simulink model "modela13"  (R2018b)
settings: Solver=VariableStepAuto  StartTime=0.0  StopTime=10.0  RelTol=1e-3
libraries: powerlib x39
settings Model: Creator=HP  LastModifiedBy=HP

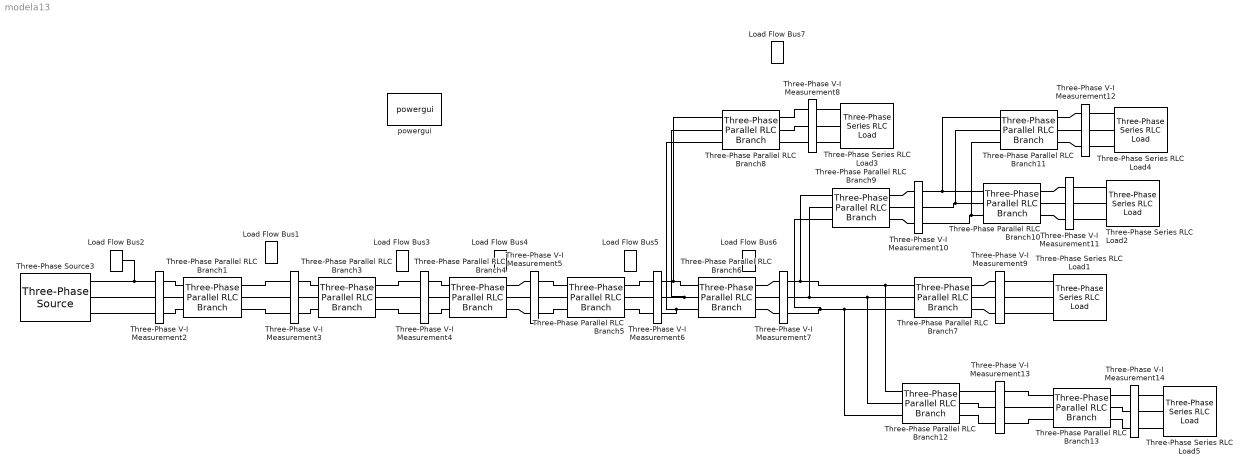
== system modela13 ==
  Load Flow Bus{1..7} (7 alike) : powerlib/Measurements/Load Flow Bus  LConnTagsString=a  Phases=single  Connectors=on one side  ID=BUS_1  Vbase=25e3  Vref=1.06  Vangle=0  VLF=1  VLFb=1  VLFc=1  angleLF=0  angleLFb=0  angleLFc=0
      settings: SourceProductName=Simscape Power Systems
  Three-Phase Parallel RLC Branch{1,3..13} (12 alike) : powerlib/Elements/Three-Phase Parallel RLC Branch  LConnTagsString=A|B|C  RConnTagsString=A|B|C  BranchType=RL  Resistance=6  Inductance=1.9e-3  Capacitance=1e-6  Measurements=None
      settings: SourceProductName=Simscape Power Systems  SourceProductBaseCode=PS
  Three-Phase Series RLC Load{1..5} (5 alike) : powerlib/Elements/Three-Phase Series RLC Load  LConnTagsString=A|B|C  Configuration=Y (grounded)  NominalVoltage=1000  Vabc=[1e3 1e3 1e3]  Vabcp=[1e3 1e3 1e3]  NominalFrequency=60  UnbalancedPower=off  ActivePower=20e6  InductivePower=10e6  CapacitivePower=0  Pabc=[10e3 9e3 11e3]  QLabc=[100 90 110]  QCabc=[100 90 110]  Pabcp=[10e3 9e3 11e3]  QLabcp=[100 90 110]  QCabcp=[100 90 110]  Measurements=None  LoadType=constant Z
  Three-Phase V-I Measurement{2..14} (13 alike) : powerlib/Measurements/Three-Phase V-I Measurement  VoltageMeasurement=no  SetLabelV=off  LabelV=Vabc  Vpu=off  VpuLL=off  CurrentMeasurement=no  SetLabelI=off  LabelI=Iabc  Ipu=off  Pbase=100e6  Vbase=500e3  OutputType=Complex  PhasorSimulation=off  PSBequivalent=0
  Three-Phase Source3 : powerlib/Electrical Sources/Three-Phase Source  InternalConnection=Yg  VoltagePhases=off  Voltage=25e3  PhaseAngle=0  Voltage_phases=[25e3 25e3 25e3]/sqrt(3)  PhaseAngles_phases=[0 -120 +120]  Frequency=50  NonIdealSource=on  SpecifyImpedance=on  Resistance=0.8929  Inductance=16.58e-3  ShortCircuitLevel=100e6  BaseVoltage=25e3  XRratio=7  BusType=swing  Pref=10e3  Qref=0  Prefabc=[10e3, 10e3, 10e3]  Qrefabc=[0, 0, 0]  Qmin=-inf  Qmax=inf
  powergui : powerlib/powergui  Priority=1  SimulationMode=Continuous  SampleTime=50e-6  frequency=60  Iterations=50  frequencyindice=50  Pbase=100e6  ErrMax=1e-4  UnitsV=kV  UnitsW=MW  buscounter=0  FunctionMessages=off  echomessages=off  EnableUseOfTLC=off  CurrentSourceSwitches=off  DisableSnubberDevices=off  DisableRonSwitches=off  DisableVfSwitches=off  DisplayEquations=off  SolverType=Tustin/Backward Euler (TBE)  Interpol=off  ExternalGateDelay=off  methode=off  Ts=100  x0status=blocks  SPID=off  SwTol=0  HookPort=off  RestoreLinks=warning  ResistiveCurrentMeasurement=off  Frange=[0:2:500]  Ylog=off  Xlog=on  ShowGrid=off  save=off  variable=ZData  structure=0  ZoomFFT=off  StartTime=0.0  cycles=1  DisplayStyle=1  fundamental=60  FreqAxis=off  MaxFrequency=1000  frequencyindicesteady=1  RmsSteady=1  display=off
  connections:
  Three-Phase V-I Measurement2/LConn2 -- Three-Phase Parallel RLC Branch1/RConn2
  Three-Phase V-I Measurement2/RConn3 -- Load Flow Bus2/LConn1 -- Three-Phase Source3/RConn3
  Three-Phase V-I Measurement2/RConn2 -- Three-Phase Source3/RConn2
  Three-Phase V-I Measurement2/RConn1 -- Three-Phase Source3/RConn1
  Three-Phase V-I Measurement2/LConn3 -- Three-Phase Parallel RLC Branch1/RConn1
  Three-Phase V-I Measurement2/LConn1 -- Three-Phase Parallel RLC Branch1/RConn3
  Three-Phase V-I Measurement3/LConn3 -- Three-Phase Parallel RLC Branch3/RConn1
  Three-Phase V-I Measurement3/LConn1 -- Three-Phase Parallel RLC Branch3/RConn3
  Three-Phase V-I Measurement3/LConn2 -- Three-Phase Parallel RLC Branch3/RConn2
  Three-Phase Parallel RLC Branch1/LConn1 -- Three-Phase V-I Measurement3/RConn3
  Three-Phase Parallel RLC Branch1/LConn2 -- Three-Phase V-I Measurement3/RConn2
  Three-Phase Parallel RLC Branch1/LConn3 -- Three-Phase V-I Measurement3/RConn1
  Three-Phase V-I Measurement4/LConn3 -- Three-Phase Parallel RLC Branch4/RConn1
  Three-Phase V-I Measurement4/LConn1 -- Three-Phase Parallel RLC Branch4/RConn3
  Three-Phase V-I Measurement4/LConn2 -- Three-Phase Parallel RLC Branch4/RConn2
  Three-Phase Parallel RLC Branch3/LConn1 -- Three-Phase V-I Measurement4/RConn3
  Three-Phase Parallel RLC Branch3/LConn2 -- Three-Phase V-I Measurement4/RConn2
  Three-Phase Parallel RLC Branch3/LConn3 -- Three-Phase V-I Measurement4/RConn1
  Three-Phase V-I Measurement5/LConn3 -- Three-Phase Parallel RLC Branch5/RConn1
  Three-Phase V-I Measurement5/LConn1 -- Three-Phase Parallel RLC Branch5/RConn3
  Three-Phase V-I Measurement5/LConn2 -- Three-Phase Parallel RLC Branch5/RConn2
  Three-Phase Parallel RLC Branch4/LConn1 -- Three-Phase V-I Measurement5/RConn3
  Three-Phase Parallel RLC Branch4/LConn2 -- Three-Phase V-I Measurement5/RConn2
  Three-Phase Parallel RLC Branch4/LConn3 -- Three-Phase V-I Measurement5/RConn1
  Three-Phase V-I Measurement6/LConn3 -- Three-Phase Parallel RLC Branch8/RConn1 -- Three-Phase Parallel RLC Branch6/RConn1
  Three-Phase V-I Measurement6/LConn1 -- Three-Phase Parallel RLC Branch6/RConn3 -- Three-Phase Parallel RLC Branch8/RConn3
  Three-Phase V-I Measurement6/LConn2 -- Three-Phase Parallel RLC Branch8/RConn2 -- Three-Phase Parallel RLC Branch6/RConn2
  Three-Phase Parallel RLC Branch5/LConn1 -- Three-Phase V-I Measurement6/RConn3
  Three-Phase Parallel RLC Branch5/LConn2 -- Three-Phase V-I Measurement6/RConn2
  Three-Phase Parallel RLC Branch5/LConn3 -- Three-Phase V-I Measurement6/RConn1
  Three-Phase V-I Measurement7/LConn3 -- Three-Phase Parallel RLC Branch9/RConn1 -- Three-Phase Parallel RLC Branch12/RConn1 -- Three-Phase Parallel RLC Branch7/RConn1
  Three-Phase V-I Measurement7/LConn1 -- Three-Phase Parallel RLC Branch9/RConn3 -- Three-Phase Parallel RLC Branch12/RConn3 -- Three-Phase Parallel RLC Branch7/RConn3
  Three-Phase V-I Measurement7/LConn2 -- Three-Phase Parallel RLC Branch9/RConn2 -- Three-Phase Parallel RLC Branch12/RConn2 -- Three-Phase Parallel RLC Branch7/RConn2
  Three-Phase Parallel RLC Branch6/LConn1 -- Three-Phase V-I Measurement7/RConn3
  Three-Phase Parallel RLC Branch6/LConn2 -- Three-Phase V-I Measurement7/RConn2
  Three-Phase Parallel RLC Branch6/LConn3 -- Three-Phase V-I Measurement7/RConn1
  Three-Phase Parallel RLC Branch8/LConn1 -- Three-Phase V-I Measurement8/RConn3
  Three-Phase Parallel RLC Branch8/LConn2 -- Three-Phase V-I Measurement8/RConn2
  Three-Phase Parallel RLC Branch8/LConn3 -- Three-Phase V-I Measurement8/RConn1
  Three-Phase Series RLC Load3/LConn1 -- Three-Phase V-I Measurement8/LConn3
  Three-Phase Series RLC Load3/LConn2 -- Three-Phase V-I Measurement8/LConn2
  Three-Phase Series RLC Load3/LConn3 -- Three-Phase V-I Measurement8/LConn1
  Three-Phase Parallel RLC Branch7/LConn1 -- Three-Phase V-I Measurement9/RConn3
  Three-Phase Parallel RLC Branch7/LConn2 -- Three-Phase V-I Measurement9/RConn2
  Three-Phase Parallel RLC Branch7/LConn3 -- Three-Phase V-I Measurement9/RConn1
  Three-Phase Series RLC Load1/LConn1 -- Three-Phase V-I Measurement9/LConn3
  Three-Phase V-I Measurement9/LConn2 -- Three-Phase Series RLC Load1/LConn2
  Three-Phase V-I Measurement9/LConn1 -- Three-Phase Series RLC Load1/LConn3
  Three-Phase Parallel RLC Branch9/LConn1 -- Three-Phase V-I Measurement10/RConn3
  Three-Phase Parallel RLC Branch9/LConn2 -- Three-Phase V-I Measurement10/RConn2
  Three-Phase Parallel RLC Branch9/LConn3 -- Three-Phase V-I Measurement10/RConn1
  Three-Phase Parallel RLC Branch10/RConn1 -- Three-Phase Parallel RLC Branch11/RConn1 -- Three-Phase V-I Measurement10/LConn3
  Three-Phase V-I Measurement10/LConn2 -- Three-Phase Parallel RLC Branch11/RConn2 -- Three-Phase Parallel RLC Branch10/RConn2
  Three-Phase V-I Measurement10/LConn1 -- Three-Phase Parallel RLC Branch11/RConn3 -- Three-Phase Parallel RLC Branch10/RConn3
  Three-Phase V-I Measurement11/RConn2 -- Three-Phase Parallel RLC Branch10/LConn2
  Three-Phase Parallel RLC Branch10/LConn1 -- Three-Phase V-I Measurement11/RConn3
  Three-Phase Parallel RLC Branch10/LConn3 -- Three-Phase V-I Measurement11/RConn1
  Three-Phase Series RLC Load2/LConn1 -- Three-Phase V-I Measurement11/LConn3
  Three-Phase Series RLC Load2/LConn2 -- Three-Phase V-I Measurement11/LConn2
  Three-Phase Series RLC Load2/LConn3 -- Three-Phase V-I Measurement11/LConn1
  Three-Phase Parallel RLC Branch11/LConn1 -- Three-Phase V-I Measurement12/RConn3
  Three-Phase Parallel RLC Branch11/LConn2 -- Three-Phase V-I Measurement12/RConn2
  Three-Phase Parallel RLC Branch11/LConn3 -- Three-Phase V-I Measurement12/RConn1
  Three-Phase Series RLC Load4/LConn1 -- Three-Phase V-I Measurement12/LConn3
  Three-Phase Series RLC Load4/LConn2 -- Three-Phase V-I Measurement12/LConn2
  Three-Phase Series RLC Load4/LConn3 -- Three-Phase V-I Measurement12/LConn1
  Three-Phase V-I Measurement13/RConn3 -- Three-Phase Parallel RLC Branch12/LConn1
  Three-Phase Parallel RLC Branch12/LConn2 -- Three-Phase V-I Measurement13/RConn2
  Three-Phase Parallel RLC Branch12/LConn3 -- Three-Phase V-I Measurement13/RConn1
  Three-Phase Parallel RLC Branch13/RConn1 -- Three-Phase V-I Measurement13/LConn3
  Three-Phase V-I Measurement13/LConn2 -- Three-Phase Parallel RLC Branch13/RConn2
  Three-Phase V-I Measurement13/LConn1 -- Three-Phase Parallel RLC Branch13/RConn3
  Three-Phase V-I Measurement14/RConn3 -- Three-Phase Parallel RLC Branch13/LConn1
  Three-Phase Parallel RLC Branch13/LConn2 -- Three-Phase V-I Measurement14/RConn2
  Three-Phase Parallel RLC Branch13/LConn3 -- Three-Phase V-I Measurement14/RConn1
  Three-Phase Series RLC Load5/LConn1 -- Three-Phase V-I Measurement14/LConn3
  Three-Phase Series RLC Load5/LConn2 -- Three-Phase V-I Measurement14/LConn2
  Three-Phase Series RLC Load5/LConn3 -- Three-Phase V-I Measurement14/LConn1
